simulink model "LQR_continous"  (R2024b)
settings: Solver=ode45  StartTime=0.0  StopTime=tsim  RelTol=1e-3  EnableMultiTasking=on
values from neighbouring files (symbols this model uses):
  A = zeros(n)    [main.m]
  B = zeros(n,1)    [main.m]    (also in point7.m)
  C = zeros(1,n)    [main.m]    (also in point7.m)
  C_state = eye(12)    [main.m]
  D_state = zeros(12, 1)    [main.m]
  K_s = lqr(A,B,Q_LQ,R_LQ)    [main.m]
  Ubar_s = inv(dcgain(Gs))*Ybar    [main.m]
  umax = +15    (= 15)    [main.m]
  umin = -15    [main.m]
  x0 = [3,0,3,0,3,0,3,0,3,0,3,0]    [main.m]
  Xbar_s = -A \ (B * Ubar_s)    [main.m]
settings Model: Creator=Administrator  LastModifiedBy=faiol
settings SolverCC: AlgebraicLoopSolver=TrustRegion
settings DataIOCC: LimitDataPoints=on  SaveFormat=Array  SignalLoggingSaveFormat=ModelDataLogs  ReturnWorkspaceOutputs=off
settings OptimizationCC: ExpressionDepthLimit=2147483647  InitFltsAndDblsToZero=on  LifeSpan=inf
settings DebuggingCC: UnderspecifiedInitializationDetection=Classic  MergeDetectMultiDrivingBlocksExec=none  SolverPrmCheckMsg=warning  FcnCallInpInsideContextMsg=warning  UnconnectedInputMsg=warning  UnconnectedOutputMsg=warning  UnconnectedLineMsg=warning  StateNameClashWarn=warning  SFUnexpectedBacktrackingDiag=warning  SFNoUnconditionalDefaultTransitionDiag=warning  SFExecutionAtInitializationDiag=none  ArithmeticOperatorsInVariantConditions=warning
settings HardwareCC: ProdBitPerPointer=32  ProdBitPerSizeT=32  ProdBitPerPtrDiffT=32  ProdLargestAtomicFloat=None  ProdIntDivRoundTo=Undefined  ProdEndianess=Unspecified  ProdWordSize=32  ProdHWDeviceType=32-bit Generic
settings ModelReferenceCC: EnableRefExpFcnMdlSchedulingChecks=on  PropagateSignalLabelsOutOfModel=off
settings SFSimCC: SimUseLocalCustomCode=off  CustomCodeUndefinedFunction=UseInterfaceOnly
settings RTWCC: RTWUseLocalCustomCode=off  GPUComputeCapability=3.5  DLArmComputeVersion=19.05
settings CodeAppCC: StateflowObjectComments=on
settings GRTTargetCC: TargetLangStandard=C89/C90 (ANSI)  CombineOutputUpdateFcns=off  GRTInterface=on
settings ConfigComp: CovMetricSettings=dw  CovSaveCumulativeToWorkspaceVar=on  CovSaveSingleToWorkspaceVar=on  CovExternalEMLEnable=off  CovSFcnEnable=off

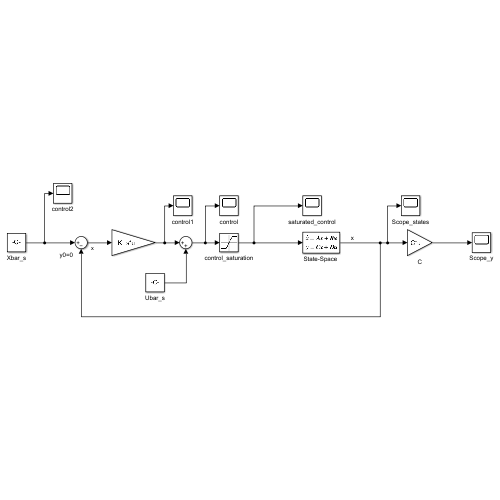
[thumbnail: Simulink's stored preview of the top-level diagram]
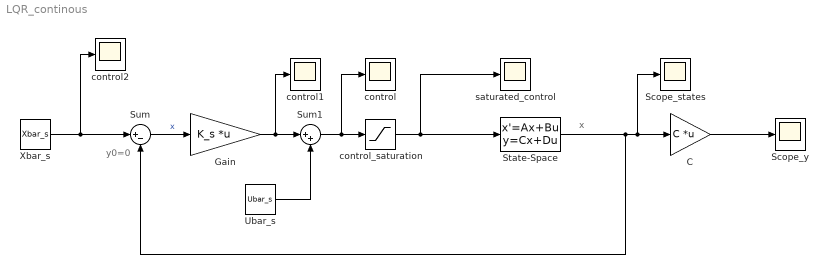
== system LQR_continous ==
  note: y0=0
  note: x
  C : Gain  Gain=C  Multiplication=Matrix(K*u)
  Gain : Gain  Gain=K_s  Multiplication=Matrix(K*u)
  Scope_states : Scope
  Scope_y : Scope
  "State-Space " : StateSpace  A=A  B=B  C=C_state  D=D_state  InitialCondition=x0  AllowTunableDMatrix=on
  Sum : Sum  Inputs=|+-
  Sum1 : Sum  Inputs=|++
  Ubar_s : Constant  Value=Ubar_s
  Xbar_s : Constant  Value=Xbar_s
  control : Scope
  control1 : Scope
  control2 : Scope
  control_saturation : Saturate  UpperLimit=umax  LowerLimit=umin
  saturated_control : Scope
  wires:
  control_saturation/1 -> "State-Space "/1, saturated_control/1
  Sum/1 -> Gain/1  "x"
  "State-Space "/1 -> Scope_states/1, C/1, Sum/2
  C/1 -> Scope_y/1
  Gain/1 -> control1/1, Sum1/1
  Sum1/1 -> control/1, control_saturation/1
  Xbar_s/1 -> control2/1, Sum/1
  Ubar_s/1 -> Sum1/2
